simulink model "ur5_simulink_ros2_pbvs_all_methods_2023b"  (R2023b)
settings: Solver=ode4  StartTime=0.0  StopTime=inf  FixedStep=0.005  RelTol=1e-3
InitFcn:
  | l=5;
model workspace (MAT data in the model file):
  SL_ROS_VariableLengthArrays_MaxSizes : object (value not decoded)
values from neighbouring files (symbols this model uses):
  D = zeros(6,12)    [ibvs_cstate.m]
undefined symbols (not defined in the file or in its folder): data, data_SL_Info, DiscIntNeverNeededParam
libraries: simulink x9, ros2lib x8, slpidlib x6, robotmaniplib x3, mpclib x3, robotcorelib x1
(part 2 of 2)

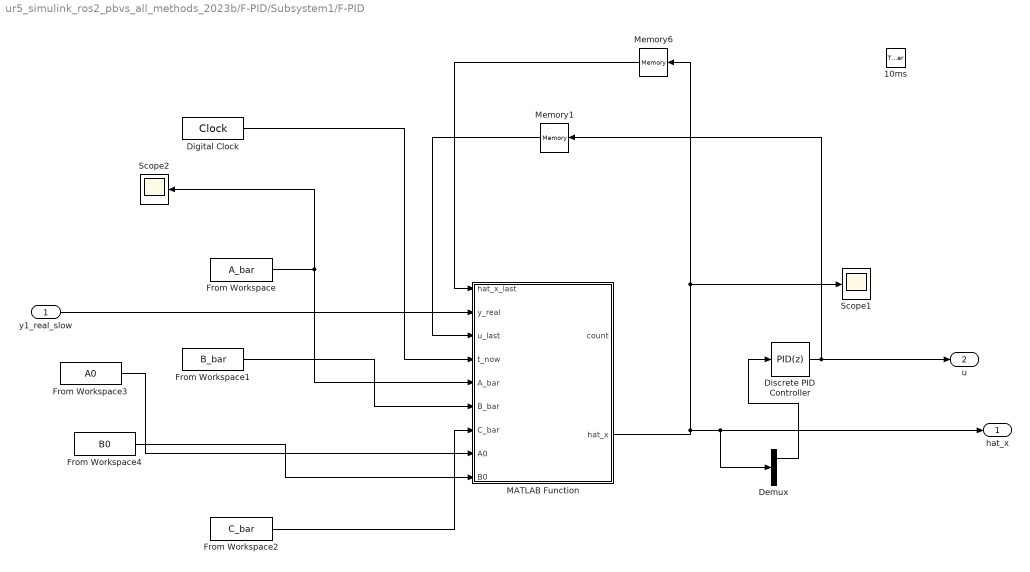
== system ur5_simulink_ros2_pbvs_all_methods_2023b/F-PID/Subsystem1/F-PID ==
  y1_real_slow : Inport
  10ms : TriggerPort  VariantControl=(inherit)  InitialTriggerSignalState=zero  PortDimensions=1
  Demux : Demux  Outputs=2
  Digital Clock : DigitalClock  SampleTime=-1
  Discrete PID Controller : slpidlib/PID Controller  Controller=PID  Form=Parallel  TimeDomain=Discrete-time  UseExternalTs=off  SampleTime=-1  IntegratorMethod=Forward Euler  FilterMethod=Forward Euler  ControllerParametersSource=internal  P=4.7  I=5  UseKiTs=off  D=0  N=100  UseFilter=on  TunerSelectOption=Transfer Function Based (PID Tuner App)  InitialConditionSource=internal  InitialConditionForIntegrator=0  InitialConditionForFilter=0  DifferentiatorICPrevScaledInput=0  ExternalReset=none  TrackingMode=off  Kt=1  LimitOutput=off  SatLimitsSource=internal  UpperSaturationLimit=inf  LowerSaturationLimit=-inf  LinearizeAsGain=off  AntiWindupMode=none  Kb=1  LimitIntegrator=off  UpperIntegratorSaturationLimit=inf  LowerIntegratorSaturationLimit=-inf  POutMin=[]  POutMax=[]  IOutMin=[]  IOutMax=[]  DOutMin=[]  DOutMax=[]  NOutMin=[]  NOutMax=[]  SumOutMin=[]  SumOutMax=[]  SaturationOutMin=[]  SaturationOutMax=[]  PParamMin=[]  PParamMax=[]  IParamMin=[]  IParamMax=[]  DParamMin=[]  DParamMax=[]  NParamMin=[]  NParamMax=[]  KbParamMin=[]  KbParamMax=[]  KtParamMin=[]  KtParamMax=[]  KbOutMin=[]  KbOutMax=[]  KtOutMin=[]  KtOutMax=[]  IntegratorOutMin=[]  IntegratorOutMax=[]  FilterOutMin=[]  FilterOutMax=[]  SumI1OutMin=[]  SumI1OutMax=[]  SumI2OutMin=[]  SumI2OutMax=[]  SumI3OutMin=[]  SumI3OutMax=[]  SumI4OutMin=[]  SumI4OutMax=[]  SumDOutMin=[]  SumDOutMax=[]  DifferentiatorOutMin=[]  DifferentiatorOutMax=[]  FilterDiffOutCoefMin=[]  FilterDiffOutCoefMax=[]  ReciprocalOutMin=[]  ReciprocalOutMax=[]  SumDenOutMin=[]  SumDenOutMax=[]  SumNumOutMin=[]  SumNumOutMax=[]  DivideOutMin=[]  DivideOutMax=[]  UdiffTsProdOutMin=[]  UdiffTsProdOutMax=[]  NTsProdOutMin=[]  NTsProdOutMax=[]  UintegralTsProdOutMin=[]  UintegralTsProdOutMax=[]  UngainTsProdOutMin=[]  UngainTsProdOutMax=[]  ClampingZeroOutDataTypeStr=Inherit: Inherit via back propagation  ClampingZeroOutMin=[]  ClampingZeroOutMax=[]  FilterDenConstantOutDataTypeStr=Inherit: Inherit via back propagation  FilterDenConstantOutMin=[]  FilterDenConstantOutMax=[]  PCopyOutDataTypeStr=Inherit: Inherit via back propagation  PCopyOutMin=[]  PCopyOutMax=[]  NCopyOutDataTypeStr=Inherit: Inherit via back propagation  NCopyOutMin=[]  NCopyOutMax=[]  IntegratorContinuousStateAttributes=''  IntegratorStateMustResolveToSignalObject=off  IntegratorRTWStateStorageClass=Auto  FilterContinuousStateAttributes=''  FilterStateMustResolveToSignalObject=off  FilterRTWStateStorageClass=Auto  ParallelPVariant=InternalParameters  IdealPVariant=Disabled  IVariant=InternalParameters  DVariant=InternalParameters  IntegratorVariant=Discrete  SatVariant=Disabled  AWVariant=Passthrough  PCopyVariant=Disabled  TRVariant=Disabled  FdbkBlocksVariant=Forward  IdealPFdbkVariant=Disabled  SatFdbkVariant=Disabled  DerivativeFilterVariant=ForwardEulerFilter  NVariant=InternalParameters  NCopyVariant=Disabled  FilterICVariant=InternalICsFilter  IntegratorICVariant=InternalICs  ExternalResetVariant=Disabled  TRSumVariant=Passthrough  SumFdbkVariant=Disabled  SumVariant=Sum_PID  TsampFilterVariant=InternalTs  TsampNgainVariant=Passthrough  TsampIntegralVariant=Disabled_SignalSpec  ExternalSaturationOutDataTypeStr=Inherit: Same as second input
      settings: LibrarySourceBlock=simulink/Discrete/Discrete PID Controller
  From Workspace : FromWorkspace  VariableName=A_bar  OutDataTypeStr=double  SampleTime=-1  OutputAfterFinalValue=Holding final value
  From Workspace1 : FromWorkspace  VariableName=B_bar  OutDataTypeStr=double  SampleTime=-1  OutputAfterFinalValue=Holding final value
  From Workspace2 : FromWorkspace  VariableName=C_bar  OutDataTypeStr=double  SampleTime=-1  OutputAfterFinalValue=Holding final value
  From Workspace3 : FromWorkspace  VariableName=A0  OutDataTypeStr=double  SampleTime=-1  OutputAfterFinalValue=Holding final value
  From Workspace4 : FromWorkspace  VariableName=B0  OutDataTypeStr=double  SampleTime=-1  OutputAfterFinalValue=Holding final value
  MATLAB Function : MATLAB Function  TreatAsAtomicUnit=on
  Memory1 : Memory  InheritSampleTime=on
  Memory6 : Memory  InheritSampleTime=on
  Scope1 : Scope
  Scope2 : Scope
  hat_x : Outport
  u : Outport  Port=2
  wires:
  From Workspace2/1 -> MATLAB Function/7(C_bar)
  From Workspace1/1 -> MATLAB Function/6(B_bar)
  Digital Clock/1 -> MATLAB Function/4(t_now)
  From Workspace/1 -> Scope2/1, MATLAB Function/5(A_bar)
  MATLAB Function/2(hat_x) -> Memory6/1, Scope1/1, Demux/1, hat_x/1
  y1_real_slow/1 -> MATLAB Function/2(y_real)
  From Workspace3/1 -> MATLAB Function/8(A0)
  From Workspace4/1 -> MATLAB Function/9(B0)
  Memory6/1 -> MATLAB Function/1(hat_x_last)
  Discrete PID Controller/1 -> Memory1/1, u/1
  Demux/1 -> Discrete PID Controller/1
  Memory1/1 -> MATLAB Function/3(u_last)

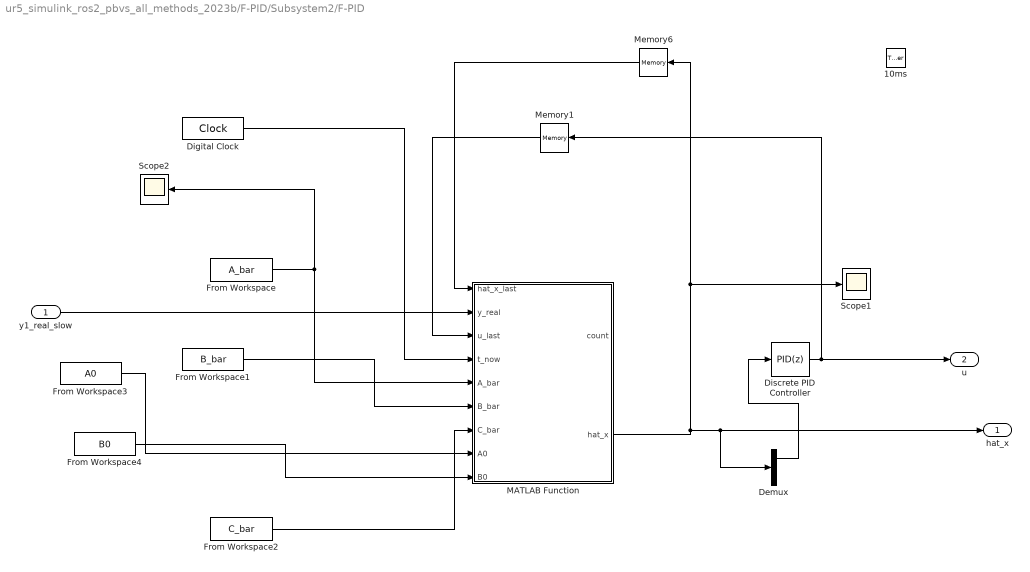
== system ur5_simulink_ros2_pbvs_all_methods_2023b/F-PID/Subsystem2/F-PID ==
  y1_real_slow : Inport
  10ms : TriggerPort  VariantControl=(inherit)  InitialTriggerSignalState=zero  PortDimensions=1
  Demux : Demux  Outputs=2
  Digital Clock : DigitalClock  SampleTime=-1
  Discrete PID Controller : slpidlib/PID Controller  Controller=PID  Form=Parallel  TimeDomain=Discrete-time  UseExternalTs=off  SampleTime=-1  IntegratorMethod=Forward Euler  FilterMethod=Forward Euler  ControllerParametersSource=internal  P=4.7  I=5  UseKiTs=off  D=0  N=100  UseFilter=on  TunerSelectOption=Transfer Function Based (PID Tuner App)  InitialConditionSource=internal  InitialConditionForIntegrator=0  InitialConditionForFilter=0  DifferentiatorICPrevScaledInput=0  ExternalReset=none  TrackingMode=off  Kt=1  LimitOutput=off  SatLimitsSource=internal  UpperSaturationLimit=inf  LowerSaturationLimit=-inf  LinearizeAsGain=off  AntiWindupMode=none  Kb=1  LimitIntegrator=off  UpperIntegratorSaturationLimit=inf  LowerIntegratorSaturationLimit=-inf  POutMin=[]  POutMax=[]  IOutMin=[]  IOutMax=[]  DOutMin=[]  DOutMax=[]  NOutMin=[]  NOutMax=[]  SumOutMin=[]  SumOutMax=[]  SaturationOutMin=[]  SaturationOutMax=[]  PParamMin=[]  PParamMax=[]  IParamMin=[]  IParamMax=[]  DParamMin=[]  DParamMax=[]  NParamMin=[]  NParamMax=[]  KbParamMin=[]  KbParamMax=[]  KtParamMin=[]  KtParamMax=[]  KbOutMin=[]  KbOutMax=[]  KtOutMin=[]  KtOutMax=[]  IntegratorOutMin=[]  IntegratorOutMax=[]  FilterOutMin=[]  FilterOutMax=[]  SumI1OutMin=[]  SumI1OutMax=[]  SumI2OutMin=[]  SumI2OutMax=[]  SumI3OutMin=[]  SumI3OutMax=[]  SumI4OutMin=[]  SumI4OutMax=[]  SumDOutMin=[]  SumDOutMax=[]  DifferentiatorOutMin=[]  DifferentiatorOutMax=[]  FilterDiffOutCoefMin=[]  FilterDiffOutCoefMax=[]  ReciprocalOutMin=[]  ReciprocalOutMax=[]  SumDenOutMin=[]  SumDenOutMax=[]  SumNumOutMin=[]  SumNumOutMax=[]  DivideOutMin=[]  DivideOutMax=[]  UdiffTsProdOutMin=[]  UdiffTsProdOutMax=[]  NTsProdOutMin=[]  NTsProdOutMax=[]  UintegralTsProdOutMin=[]  UintegralTsProdOutMax=[]  UngainTsProdOutMin=[]  UngainTsProdOutMax=[]  ClampingZeroOutDataTypeStr=Inherit: Inherit via back propagation  ClampingZeroOutMin=[]  ClampingZeroOutMax=[]  FilterDenConstantOutDataTypeStr=Inherit: Inherit via back propagation  FilterDenConstantOutMin=[]  FilterDenConstantOutMax=[]  PCopyOutDataTypeStr=Inherit: Inherit via back propagation  PCopyOutMin=[]  PCopyOutMax=[]  NCopyOutDataTypeStr=Inherit: Inherit via back propagation  NCopyOutMin=[]  NCopyOutMax=[]  IntegratorContinuousStateAttributes=''  IntegratorStateMustResolveToSignalObject=off  IntegratorRTWStateStorageClass=Auto  FilterContinuousStateAttributes=''  FilterStateMustResolveToSignalObject=off  FilterRTWStateStorageClass=Auto  ParallelPVariant=InternalParameters  IdealPVariant=Disabled  IVariant=InternalParameters  DVariant=InternalParameters  IntegratorVariant=Discrete  SatVariant=Disabled  AWVariant=Passthrough  PCopyVariant=Disabled  TRVariant=Disabled  FdbkBlocksVariant=Forward  IdealPFdbkVariant=Disabled  SatFdbkVariant=Disabled  DerivativeFilterVariant=ForwardEulerFilter  NVariant=InternalParameters  NCopyVariant=Disabled  FilterICVariant=InternalICsFilter  IntegratorICVariant=InternalICs  ExternalResetVariant=Disabled  TRSumVariant=Passthrough  SumFdbkVariant=Disabled  SumVariant=Sum_PID  TsampFilterVariant=InternalTs  TsampNgainVariant=Passthrough  TsampIntegralVariant=Disabled_SignalSpec  ExternalSaturationOutDataTypeStr=Inherit: Same as second input
      settings: LibrarySourceBlock=simulink/Discrete/Discrete PID Controller
  From Workspace : FromWorkspace  VariableName=A_bar  OutDataTypeStr=double  SampleTime=-1  OutputAfterFinalValue=Holding final value
  From Workspace1 : FromWorkspace  VariableName=B_bar  OutDataTypeStr=double  SampleTime=-1  OutputAfterFinalValue=Holding final value
  From Workspace2 : FromWorkspace  VariableName=C_bar  OutDataTypeStr=double  SampleTime=-1  OutputAfterFinalValue=Holding final value
  From Workspace3 : FromWorkspace  VariableName=A0  OutDataTypeStr=double  SampleTime=-1  OutputAfterFinalValue=Holding final value
  From Workspace4 : FromWorkspace  VariableName=B0  OutDataTypeStr=double  SampleTime=-1  OutputAfterFinalValue=Holding final value
  MATLAB Function : MATLAB Function  TreatAsAtomicUnit=on
  Memory1 : Memory  InheritSampleTime=on
  Memory6 : Memory  InheritSampleTime=on
  Scope1 : Scope
  Scope2 : Scope
  hat_x : Outport
  u : Outport  Port=2
  wires:
  From Workspace2/1 -> MATLAB Function/7(C_bar)
  From Workspace1/1 -> MATLAB Function/6(B_bar)
  Digital Clock/1 -> MATLAB Function/4(t_now)
  From Workspace/1 -> Scope2/1, MATLAB Function/5(A_bar)
  MATLAB Function/2(hat_x) -> Memory6/1, Scope1/1, Demux/1, hat_x/1
  y1_real_slow/1 -> MATLAB Function/2(y_real)
  From Workspace3/1 -> MATLAB Function/8(A0)
  From Workspace4/1 -> MATLAB Function/9(B0)
  Memory6/1 -> MATLAB Function/1(hat_x_last)
  Discrete PID Controller/1 -> Memory1/1, u/1
  Demux/1 -> Discrete PID Controller/1
  Memory1/1 -> MATLAB Function/3(u_last)

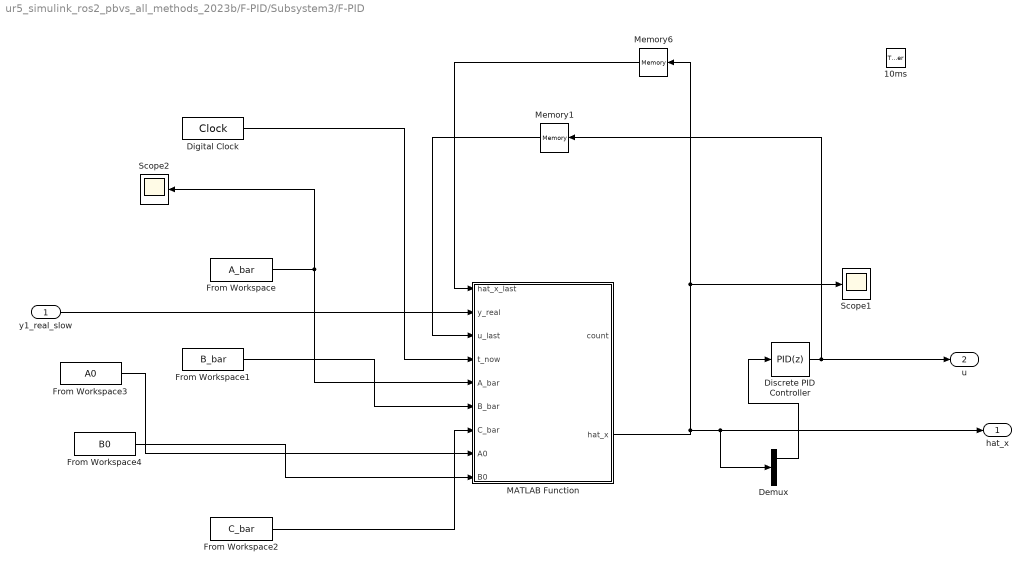
== system ur5_simulink_ros2_pbvs_all_methods_2023b/F-PID/Subsystem3/F-PID ==
  y1_real_slow : Inport
  10ms : TriggerPort  VariantControl=(inherit)  InitialTriggerSignalState=zero  PortDimensions=1
  Demux : Demux  Outputs=2
  Digital Clock : DigitalClock  SampleTime=-1
  Discrete PID Controller : slpidlib/PID Controller  Controller=PID  Form=Parallel  TimeDomain=Discrete-time  UseExternalTs=off  SampleTime=-1  IntegratorMethod=Forward Euler  FilterMethod=Forward Euler  ControllerParametersSource=internal  P=4.7  I=5  UseKiTs=off  D=0  N=100  UseFilter=on  TunerSelectOption=Transfer Function Based (PID Tuner App)  InitialConditionSource=internal  InitialConditionForIntegrator=0  InitialConditionForFilter=0  DifferentiatorICPrevScaledInput=0  ExternalReset=none  TrackingMode=off  Kt=1  LimitOutput=off  SatLimitsSource=internal  UpperSaturationLimit=inf  LowerSaturationLimit=-inf  LinearizeAsGain=off  AntiWindupMode=none  Kb=1  LimitIntegrator=off  UpperIntegratorSaturationLimit=inf  LowerIntegratorSaturationLimit=-inf  POutMin=[]  POutMax=[]  IOutMin=[]  IOutMax=[]  DOutMin=[]  DOutMax=[]  NOutMin=[]  NOutMax=[]  SumOutMin=[]  SumOutMax=[]  SaturationOutMin=[]  SaturationOutMax=[]  PParamMin=[]  PParamMax=[]  IParamMin=[]  IParamMax=[]  DParamMin=[]  DParamMax=[]  NParamMin=[]  NParamMax=[]  KbParamMin=[]  KbParamMax=[]  KtParamMin=[]  KtParamMax=[]  KbOutMin=[]  KbOutMax=[]  KtOutMin=[]  KtOutMax=[]  IntegratorOutMin=[]  IntegratorOutMax=[]  FilterOutMin=[]  FilterOutMax=[]  SumI1OutMin=[]  SumI1OutMax=[]  SumI2OutMin=[]  SumI2OutMax=[]  SumI3OutMin=[]  SumI3OutMax=[]  SumI4OutMin=[]  SumI4OutMax=[]  SumDOutMin=[]  SumDOutMax=[]  DifferentiatorOutMin=[]  DifferentiatorOutMax=[]  FilterDiffOutCoefMin=[]  FilterDiffOutCoefMax=[]  ReciprocalOutMin=[]  ReciprocalOutMax=[]  SumDenOutMin=[]  SumDenOutMax=[]  SumNumOutMin=[]  SumNumOutMax=[]  DivideOutMin=[]  DivideOutMax=[]  UdiffTsProdOutMin=[]  UdiffTsProdOutMax=[]  NTsProdOutMin=[]  NTsProdOutMax=[]  UintegralTsProdOutMin=[]  UintegralTsProdOutMax=[]  UngainTsProdOutMin=[]  UngainTsProdOutMax=[]  ClampingZeroOutDataTypeStr=Inherit: Inherit via back propagation  ClampingZeroOutMin=[]  ClampingZeroOutMax=[]  FilterDenConstantOutDataTypeStr=Inherit: Inherit via back propagation  FilterDenConstantOutMin=[]  FilterDenConstantOutMax=[]  PCopyOutDataTypeStr=Inherit: Inherit via back propagation  PCopyOutMin=[]  PCopyOutMax=[]  NCopyOutDataTypeStr=Inherit: Inherit via back propagation  NCopyOutMin=[]  NCopyOutMax=[]  IntegratorContinuousStateAttributes=''  IntegratorStateMustResolveToSignalObject=off  IntegratorRTWStateStorageClass=Auto  FilterContinuousStateAttributes=''  FilterStateMustResolveToSignalObject=off  FilterRTWStateStorageClass=Auto  ParallelPVariant=InternalParameters  IdealPVariant=Disabled  IVariant=InternalParameters  DVariant=InternalParameters  IntegratorVariant=Discrete  SatVariant=Disabled  AWVariant=Passthrough  PCopyVariant=Disabled  TRVariant=Disabled  FdbkBlocksVariant=Forward  IdealPFdbkVariant=Disabled  SatFdbkVariant=Disabled  DerivativeFilterVariant=ForwardEulerFilter  NVariant=InternalParameters  NCopyVariant=Disabled  FilterICVariant=InternalICsFilter  IntegratorICVariant=InternalICs  ExternalResetVariant=Disabled  TRSumVariant=Passthrough  SumFdbkVariant=Disabled  SumVariant=Sum_PID  TsampFilterVariant=InternalTs  TsampNgainVariant=Passthrough  TsampIntegralVariant=Disabled_SignalSpec  ExternalSaturationOutDataTypeStr=Inherit: Same as second input
      settings: LibrarySourceBlock=simulink/Discrete/Discrete PID Controller
  From Workspace : FromWorkspace  VariableName=A_bar  OutDataTypeStr=double  SampleTime=-1  OutputAfterFinalValue=Holding final value
  From Workspace1 : FromWorkspace  VariableName=B_bar  OutDataTypeStr=double  SampleTime=-1  OutputAfterFinalValue=Holding final value
  From Workspace2 : FromWorkspace  VariableName=C_bar  OutDataTypeStr=double  SampleTime=-1  OutputAfterFinalValue=Holding final value
  From Workspace3 : FromWorkspace  VariableName=A0  OutDataTypeStr=double  SampleTime=-1  OutputAfterFinalValue=Holding final value
  From Workspace4 : FromWorkspace  VariableName=B0  OutDataTypeStr=double  SampleTime=-1  OutputAfterFinalValue=Holding final value
  MATLAB Function : MATLAB Function  TreatAsAtomicUnit=on
  Memory1 : Memory  InheritSampleTime=on
  Memory6 : Memory  InheritSampleTime=on
  Scope1 : Scope
  Scope2 : Scope
  hat_x : Outport
  u : Outport  Port=2
  wires:
  From Workspace2/1 -> MATLAB Function/7(C_bar)
  From Workspace1/1 -> MATLAB Function/6(B_bar)
  Digital Clock/1 -> MATLAB Function/4(t_now)
  From Workspace/1 -> Scope2/1, MATLAB Function/5(A_bar)
  MATLAB Function/2(hat_x) -> Memory6/1, Scope1/1, Demux/1, hat_x/1
  y1_real_slow/1 -> MATLAB Function/2(y_real)
  From Workspace3/1 -> MATLAB Function/8(A0)
  From Workspace4/1 -> MATLAB Function/9(B0)
  Memory6/1 -> MATLAB Function/1(hat_x_last)
  Discrete PID Controller/1 -> Memory1/1, u/1
  Demux/1 -> Discrete PID Controller/1
  Memory1/1 -> MATLAB Function/3(u_last)

== system ur5_simulink_ros2_pbvs_all_methods_2023b/MPC-DOB/mpc/Subsystem ==
  ex : Inport
  u : Inport  Port=2
  Trigger : TriggerPort  VariantControl=(inherit)  PortDimensions=1
  Scope : Scope
  Scope5 : Scope
  dob : Subsystem
  dhat : Outport
  wires:
  ex/1 -> Scope/1, dob/1(ex)
  dob/1(dhat) -> dhat/1, Scope5/1
  u/1 -> dob/2(u)

== system ur5_simulink_ros2_pbvs_all_methods_2023b/MPC-DOB/mpc1/Subsystem ==
  ex : Inport
  u : Inport  Port=2
  Trigger : TriggerPort  VariantControl=(inherit)  PortDimensions=1
  Scope : Scope
  Scope5 : Scope
  dob : Subsystem
  dhat : Outport
  wires:
  ex/1 -> Scope/1, dob/1(ex)
  dob/1(dhat) -> dhat/1, Scope5/1
  u/1 -> dob/2(u)

== system ur5_simulink_ros2_pbvs_all_methods_2023b/MPC-DOB/mpc2/Subsystem ==
  ex : Inport
  u : Inport  Port=2
  Trigger : TriggerPort  VariantControl=(inherit)  PortDimensions=1
  Scope : Scope
  Scope5 : Scope
  dob : Subsystem
  dhat : Outport
  wires:
  ex/1 -> Scope/1, dob/1(ex)
  dob/1(dhat) -> dhat/1, Scope5/1
  u/1 -> dob/2(u)

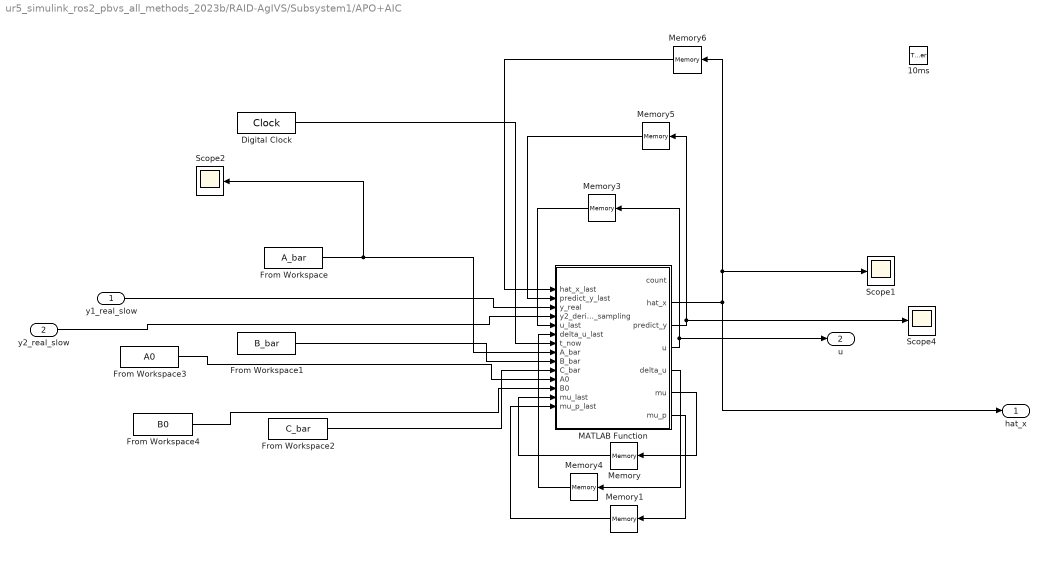
== system ur5_simulink_ros2_pbvs_all_methods_2023b/RAID-AgIVS/Subsystem1/APO+AIC ==
  y1_real_slow : Inport
  y2_real_slow : Inport  Port=2
  10ms : TriggerPort  VariantControl=(inherit)  InitialTriggerSignalState=zero  PortDimensions=1
  Digital Clock : DigitalClock  SampleTime=-1
  From Workspace : FromWorkspace  VariableName=A_bar  OutDataTypeStr=double  SampleTime=-1  OutputAfterFinalValue=Holding final value
  From Workspace1 : FromWorkspace  VariableName=B_bar  OutDataTypeStr=double  SampleTime=-1  OutputAfterFinalValue=Holding final value
  From Workspace2 : FromWorkspace  VariableName=C_bar  OutDataTypeStr=double  SampleTime=-1  OutputAfterFinalValue=Holding final value
  From Workspace3 : FromWorkspace  VariableName=A0  OutDataTypeStr=double  SampleTime=-1  OutputAfterFinalValue=Holding final value
  From Workspace4 : FromWorkspace  VariableName=B0  OutDataTypeStr=double  SampleTime=-1  OutputAfterFinalValue=Holding final value
  MATLAB Function : MATLAB Function  TreatAsAtomicUnit=on
  Memory{,1,3..6} (6 alike) : Memory  InheritSampleTime=on
  Scope1 : Scope
  Scope2 : Scope
  Scope4 : Scope
  hat_x : Outport
  u : Outport  Port=2
  wires:
  From Workspace2/1 -> MATLAB Function/10(C_bar)
  From Workspace1/1 -> MATLAB Function/9(B_bar)
  Digital Clock/1 -> MATLAB Function/7(t_now)
  Memory5/1 -> MATLAB Function/2(predict_y_last)
  MATLAB Function/3(predict_y) -> Memory5/1, Scope4/1
  From Workspace/1 -> Scope2/1, MATLAB Function/8(A_bar)
  MATLAB Function/2(hat_x) -> Memory6/1, Scope1/1, hat_x/1
  y1_real_slow/1 -> MATLAB Function/3(y_real)
  From Workspace3/1 -> MATLAB Function/11(A0)
  From Workspace4/1 -> MATLAB Function/12(B0)
  MATLAB Function/6(mu) -> Memory/1
  Memory/1 -> MATLAB Function/13(mu_last)
  MATLAB Function/7(mu_p) -> Memory1/1
  Memory1/1 -> MATLAB Function/14(mu_p_last)
  y2_real_slow/1 -> MATLAB Function/4(y2_derivative_sampling)
  MATLAB Function/4(u) -> Memory3/1, u/1
  Memory3/1 -> MATLAB Function/5(u_last)
  MATLAB Function/5(delta_u) -> Memory4/1
  Memory6/1 -> MATLAB Function/1(hat_x_last)
  Memory4/1 -> MATLAB Function/6(delta_u_last)

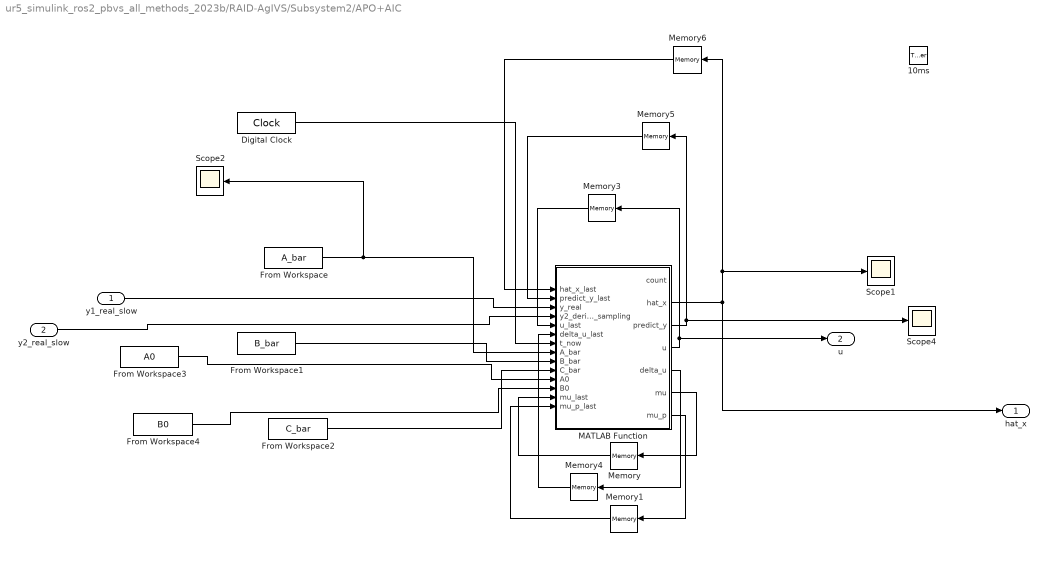
== system ur5_simulink_ros2_pbvs_all_methods_2023b/RAID-AgIVS/Subsystem2/APO+AIC ==
  y1_real_slow : Inport
  y2_real_slow : Inport  Port=2
  10ms : TriggerPort  VariantControl=(inherit)  InitialTriggerSignalState=zero  PortDimensions=1
  Digital Clock : DigitalClock  SampleTime=-1
  From Workspace : FromWorkspace  VariableName=A_bar  OutDataTypeStr=double  SampleTime=-1  OutputAfterFinalValue=Holding final value
  From Workspace1 : FromWorkspace  VariableName=B_bar  OutDataTypeStr=double  SampleTime=-1  OutputAfterFinalValue=Holding final value
  From Workspace2 : FromWorkspace  VariableName=C_bar  OutDataTypeStr=double  SampleTime=-1  OutputAfterFinalValue=Holding final value
  From Workspace3 : FromWorkspace  VariableName=A0  OutDataTypeStr=double  SampleTime=-1  OutputAfterFinalValue=Holding final value
  From Workspace4 : FromWorkspace  VariableName=B0  OutDataTypeStr=double  SampleTime=-1  OutputAfterFinalValue=Holding final value
  MATLAB Function : MATLAB Function  TreatAsAtomicUnit=on
  Memory{,1,3..6} (6 alike) : Memory  InheritSampleTime=on
  Scope1 : Scope
  Scope2 : Scope
  Scope4 : Scope
  hat_x : Outport
  u : Outport  Port=2
  wires:
  From Workspace2/1 -> MATLAB Function/10(C_bar)
  From Workspace1/1 -> MATLAB Function/9(B_bar)
  Digital Clock/1 -> MATLAB Function/7(t_now)
  Memory5/1 -> MATLAB Function/2(predict_y_last)
  MATLAB Function/3(predict_y) -> Memory5/1, Scope4/1
  From Workspace/1 -> Scope2/1, MATLAB Function/8(A_bar)
  MATLAB Function/2(hat_x) -> Memory6/1, Scope1/1, hat_x/1
  y1_real_slow/1 -> MATLAB Function/3(y_real)
  From Workspace3/1 -> MATLAB Function/11(A0)
  From Workspace4/1 -> MATLAB Function/12(B0)
  MATLAB Function/6(mu) -> Memory/1
  Memory/1 -> MATLAB Function/13(mu_last)
  MATLAB Function/7(mu_p) -> Memory1/1
  Memory1/1 -> MATLAB Function/14(mu_p_last)
  y2_real_slow/1 -> MATLAB Function/4(y2_derivative_sampling)
  MATLAB Function/4(u) -> Memory3/1, u/1
  Memory3/1 -> MATLAB Function/5(u_last)
  MATLAB Function/5(delta_u) -> Memory4/1
  Memory6/1 -> MATLAB Function/1(hat_x_last)
  Memory4/1 -> MATLAB Function/6(delta_u_last)

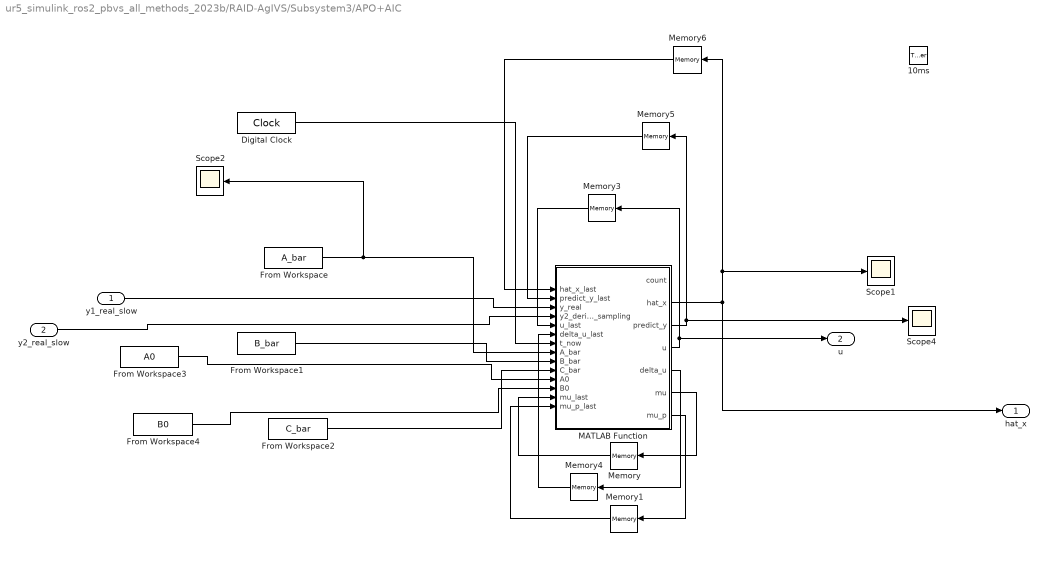
== system ur5_simulink_ros2_pbvs_all_methods_2023b/RAID-AgIVS/Subsystem3/APO+AIC ==
  y1_real_slow : Inport
  y2_real_slow : Inport  Port=2
  10ms : TriggerPort  VariantControl=(inherit)  InitialTriggerSignalState=zero  PortDimensions=1
  Digital Clock : DigitalClock  SampleTime=-1
  From Workspace : FromWorkspace  VariableName=A_bar  OutDataTypeStr=double  SampleTime=-1  OutputAfterFinalValue=Holding final value
  From Workspace1 : FromWorkspace  VariableName=B_bar  OutDataTypeStr=double  SampleTime=-1  OutputAfterFinalValue=Holding final value
  From Workspace2 : FromWorkspace  VariableName=C_bar  OutDataTypeStr=double  SampleTime=-1  OutputAfterFinalValue=Holding final value
  From Workspace3 : FromWorkspace  VariableName=A0  OutDataTypeStr=double  SampleTime=-1  OutputAfterFinalValue=Holding final value
  From Workspace4 : FromWorkspace  VariableName=B0  OutDataTypeStr=double  SampleTime=-1  OutputAfterFinalValue=Holding final value
  MATLAB Function : MATLAB Function  TreatAsAtomicUnit=on
  Memory{,1,3..6} (6 alike) : Memory  InheritSampleTime=on
  Scope1 : Scope
  Scope2 : Scope
  Scope4 : Scope
  hat_x : Outport
  u : Outport  Port=2
  wires:
  From Workspace2/1 -> MATLAB Function/10(C_bar)
  From Workspace1/1 -> MATLAB Function/9(B_bar)
  Digital Clock/1 -> MATLAB Function/7(t_now)
  Memory5/1 -> MATLAB Function/2(predict_y_last)
  MATLAB Function/3(predict_y) -> Memory5/1, Scope4/1
  From Workspace/1 -> Scope2/1, MATLAB Function/8(A_bar)
  MATLAB Function/2(hat_x) -> Memory6/1, Scope1/1, hat_x/1
  y1_real_slow/1 -> MATLAB Function/3(y_real)
  From Workspace3/1 -> MATLAB Function/11(A0)
  From Workspace4/1 -> MATLAB Function/12(B0)
  MATLAB Function/6(mu) -> Memory/1
  Memory/1 -> MATLAB Function/13(mu_last)
  MATLAB Function/7(mu_p) -> Memory1/1
  Memory1/1 -> MATLAB Function/14(mu_p_last)
  y2_real_slow/1 -> MATLAB Function/4(y2_derivative_sampling)
  MATLAB Function/4(u) -> Memory3/1, u/1
  Memory3/1 -> MATLAB Function/5(u_last)
  MATLAB Function/5(delta_u) -> Memory4/1
  Memory6/1 -> MATLAB Function/1(hat_x_last)
  Memory4/1 -> MATLAB Function/6(delta_u_last)

== system ur5_simulink_ros2_pbvs_all_methods_2023b/MPC-DOB/mpc/Subsystem/dob ==
  ex : Inport
  u : Inport  Port=2
  Add3 : Sum
  Add4 : Sum  Inputs=+-
  Discrete-Time Integrator : DiscreteIntegrator  SampleTime=-1  LimitOutput=on  UpperSaturationLimit=5  LowerSaturationLimit=-5  ICPrevOutput=DiscIntNeverNeededParam  ICPrevScaledInput=DiscIntNeverNeededParam
  Gain1 : Gain  Gain=-l
  Gain2 : Gain  Gain=l
  dhat : Outport
  wires:
  Gain1/1 -> Discrete-Time Integrator/1
  Add4/1 -> Gain1/1
  Add3/1 -> dhat/1, Add4/1
  Gain2/1 -> Add3/1
  Discrete-Time Integrator/1 -> Add3/2
  ex/1 -> Gain2/1
  u/1 -> Add4/2

== system ur5_simulink_ros2_pbvs_all_methods_2023b/MPC-DOB/mpc1/Subsystem/dob ==
  ex : Inport
  u : Inport  Port=2
  Add3 : Sum
  Add4 : Sum  Inputs=+-
  Discrete-Time Integrator : DiscreteIntegrator  SampleTime=-1  LimitOutput=on  UpperSaturationLimit=5  LowerSaturationLimit=-5  ICPrevOutput=DiscIntNeverNeededParam  ICPrevScaledInput=DiscIntNeverNeededParam
  Gain1 : Gain  Gain=-l
  Gain2 : Gain  Gain=l
  dhat : Outport
  wires:
  Gain1/1 -> Discrete-Time Integrator/1
  Add4/1 -> Gain1/1
  Add3/1 -> dhat/1, Add4/1
  Gain2/1 -> Add3/1
  Discrete-Time Integrator/1 -> Add3/2
  ex/1 -> Gain2/1
  u/1 -> Add4/2

== system ur5_simulink_ros2_pbvs_all_methods_2023b/MPC-DOB/mpc2/Subsystem/dob ==
  ex : Inport
  u : Inport  Port=2
  Add3 : Sum
  Add4 : Sum  Inputs=+-
  Discrete-Time Integrator : DiscreteIntegrator  SampleTime=-1  LimitOutput=on  UpperSaturationLimit=5  LowerSaturationLimit=-5  ICPrevOutput=DiscIntNeverNeededParam  ICPrevScaledInput=DiscIntNeverNeededParam
  Gain1 : Gain  Gain=-l
  Gain2 : Gain  Gain=l
  dhat : Outport
  wires:
  Gain1/1 -> Discrete-Time Integrator/1
  Add4/1 -> Gain1/1
  Add3/1 -> dhat/1, Add4/1
  Gain2/1 -> Add3/1
  Discrete-Time Integrator/1 -> Add3/2
  ex/1 -> Gain2/1
  u/1 -> Add4/2

== matlab function ur5_simulink_ros2_pbvs_all_methods_2023b/F-PID/Subsystem1/F-PID/MATLAB Function ==
  data: count output; hat_x_last input; y_real input; u_last input; hat_x output; t_now input; A_bar input; B_bar input; C_bar input; A0 input; B0 input
function [count, hat_x] = fcn(hat_x_last, y_real, u_last, t_now,A_bar,B_bar,C_bar,A0,B0)
if(t_now==0)
    count=0;
    hat_x = zeros(2,1);
    hat_x(1,1)=y_real;
else
    count=mod(t_now,0.05);
    if(count==0)%在采样的时刻
        hat_x=A_bar*hat_x_last +B_bar*u_last+ C_bar*y_real;
    else%在两个采样时刻之间
        hat_x = A0*hat_x_last+B0*u_last;
    end
end
end

% function [count,hat_x,predict_y, u, delta_u, mu, mu_p, mu_pp] = fcn(hat_x_last, predict_y_last, y_real,y2_derivative_sampling,y3_real_slow, u_last,delta_u_last,t_now,A_bar,B_bar,C_bar,A0,B0,mu_last, mu_p_last, mu_pp_last)
% if(t_now==0)
%     count=0;
%     hat_x = zeros(3,1);
%     predict_y = y_real;
%     hat_x(1,1)=y_real;
%     u_now=0;
%     hat_x = A_bar*hat_x + B_bar*u_now+ C_bar*predict_y;
%     [u, delta_u, mu, mu_p, mu_pp]  = AIC3(t_now, 1, y_real,hat_x(1,1),y2_derivative_sampling,hat_x(2,1), y3_real_slow, hat_x(3,1), mu_last, mu_p_last, mu_pp_last, u_last);
%     %predict_y=[1 0 0]*(A0*hat_x+B0*delta_u); 
%     
% else
%     count=mod(t_now,0.05);
%     if(count==0)%在采样的时刻
%         predict_y=y_real;
%         hat_x=A_bar*hat_x_last +B_bar*delta_u_last+ C_bar*predict_y;
%         %hat_x(1,1)=y_real;
%         [u, delta_u, mu, mu_p, mu_pp]  = AIC3(t_now, 1, y_real,hat_x(1,1),y2_derivative_sampling,hat_x(2,1), y3_real_slow, hat_x(3,1), mu_last, mu_p_last, mu_pp_last, u_last);
% 
%         %predict_y=[1 0 0]*(A0*hat_x+B0*delta_u);
%         
%     else%在两个采样时刻之间
%         predict_y=[1 0 0]*(A0*hat_x_last+B0*delta_u_last);
%         hat_x=A_bar*hat_x_last + B_bar*delta_u_last+C_bar*predict_y_last;
%         [u, delta_u, mu, mu_p, mu_pp]  = AIC3(t_now, 1, y_real,hat_x(1,1),y2_derivative_sampling,hat_x(2,1), y3_real_slow, hat_x(3,1), mu_last, mu_p_last, mu_pp_last, u_last);
%         %predict_y=[1 0 0]*(A0*hat_x+B0*delta_u);
%         
%     end
% end
% end

== matlab function ur5_simulink_ros2_pbvs_all_methods_2023b/F-PID/Subsystem2/F-PID/MATLAB Function ==
  data: count output; hat_x_last input; y_real input; u_last input; hat_x output; t_now input; A_bar input; B_bar input; C_bar input; A0 input; B0 input
function [count, hat_x] = fcn(hat_x_last, y_real, u_last, t_now,A_bar,B_bar,C_bar,A0,B0)
if(t_now==0)
    count=0;
    hat_x = zeros(2,1);
    hat_x(1,1)=y_real;
else
    count=mod(t_now,0.05);
    if(count==0)%在采样的时刻
        hat_x=A_bar*hat_x_last +B_bar*u_last+ C_bar*y_real;
    else%在两个采样时刻之间
        hat_x = A0*hat_x_last+B0*u_last;
    end
end
end

% function [count,hat_x,predict_y, u, delta_u, mu, mu_p, mu_pp] = fcn(hat_x_last, predict_y_last, y_real,y2_derivative_sampling,y3_real_slow, u_last,delta_u_last,t_now,A_bar,B_bar,C_bar,A0,B0,mu_last, mu_p_last, mu_pp_last)
% if(t_now==0)
%     count=0;
%     hat_x = zeros(3,1);
%     predict_y = y_real;
%     hat_x(1,1)=y_real;
%     u_now=0;
%     hat_x = A_bar*hat_x + B_bar*u_now+ C_bar*predict_y;
%     [u, delta_u, mu, mu_p, mu_pp]  = AIC3(t_now, 1, y_real,hat_x(1,1),y2_derivative_sampling,hat_x(2,1), y3_real_slow, hat_x(3,1), mu_last, mu_p_last, mu_pp_last, u_last);
%     %predict_y=[1 0 0]*(A0*hat_x+B0*delta_u); 
%     
% else
%     count=mod(t_now,0.05);
%     if(count==0)%在采样的时刻
%         predict_y=y_real;
%         hat_x=A_bar*hat_x_last +B_bar*delta_u_last+ C_bar*predict_y;
%         %hat_x(1,1)=y_real;
%         [u, delta_u, mu, mu_p, mu_pp]  = AIC3(t_now, 1, y_real,hat_x(1,1),y2_derivative_sampling,hat_x(2,1), y3_real_slow, hat_x(3,1), mu_last, mu_p_last, mu_pp_last, u_last);
% 
%         %predict_y=[1 0 0]*(A0*hat_x+B0*delta_u);
%         
%     else%在两个采样时刻之间
%         predict_y=[1 0 0]*(A0*hat_x_last+B0*delta_u_last);
%         hat_x=A_bar*hat_x_last + B_bar*delta_u_last+C_bar*predict_y_last;
%         [u, delta_u, mu, mu_p, mu_pp]  = AIC3(t_now, 1, y_real,hat_x(1,1),y2_derivative_sampling,hat_x(2,1), y3_real_slow, hat_x(3,1), mu_last, mu_p_last, mu_pp_last, u_last);
%         %predict_y=[1 0 0]*(A0*hat_x+B0*delta_u);
%         
%     end
% end
% end

== matlab function ur5_simulink_ros2_pbvs_all_methods_2023b/MATLAB Function3 ==
  data: camera_rot input; obj_pos input; y output
function y = fcn(camera_rot, obj_pos)
    temp_pos = [obj_pos(1);obj_pos(2);obj_pos(3);1];
    new_pos = camera_rot*temp_pos;
    y = new_pos(1:3);
end

== matlab function ur5_simulink_ros2_pbvs_all_methods_2023b/joint vel to ros3/to ros2 ==
  data: u input; flag input; y output; joint1 input; joint2 input; joint3 input; joint4 input; joint5 input; joint6 input
function y  = fcn(u,flag, joint1, joint2, joint3, joint4, joint5, joint6)
    y = zeros(128,1);
    if(flag==0)
        y(1) = u(1);
        y(2) = u(2);
        y(3) = u(3);
        y(4) = u(4);
        y(5) = u(5);
        y(6) = u(6);
    else
        y(1) = joint1;
        y(2) = joint2;
        y(3) = joint3;
        y(4) = joint4;
        y(5) = joint5;
        y(6) = joint6;
    end
end

== matlab function ur5_simulink_ros2_pbvs_all_methods_2023b/RAID-AgIVS/Subsystem1/APO+AIC/MATLAB Function ==
  data: count output; hat_x_last input; predict_y_last input; y_real input; y2_derivative_sampling input; u_last input; delta_u_last input; hat_x output; t_now input; A_bar input; B_bar input; C_bar input; predict_y output; A0 input; B0 input; mu_last input; mu_p_last input; u output; delta_u output; mu output; mu_p output
function [count,hat_x,predict_y, u, delta_u, mu, mu_p] = fcn(hat_x_last, predict_y_last, y_real,y2_derivative_sampling, u_last,delta_u_last,t_now,A_bar,B_bar,C_bar,A0,B0,mu_last, mu_p_last)
if(t_now==0)
    count=0;
    hat_x = zeros(2,1);
    predict_y = y_real;
    hat_x(1,1)=y_real;
    [u, delta_u, mu, mu_p]  = AIC2(t_now, 1, y_real,hat_x(1,1),y2_derivative_sampling,hat_x(2,1), mu_last, mu_p_last, u_last);
else
    count=mod(t_now,0.05);
    if(count==0)%在采样的时刻
        predict_y=y_real;
        hat_x=A_bar*hat_x_last +B_bar*delta_u_last/0.01+ C_bar*predict_y;
        [u, delta_u, mu, mu_p]  = AIC2(t_now, 1, y_real,hat_x(1,1),y2_derivative_sampling,hat_x(2,1), mu_last, mu_p_last, u_last);
    else%在两个采样时刻之间
        predict_y=[1 0]*(A0*hat_x_last+B0*delta_u_last);
        hat_x=A_bar*hat_x_last + B_bar*delta_u_last/0.01+C_bar*predict_y_last;
        [u, delta_u, mu, mu_p]  = AIC2(t_now, 1, y_real,hat_x(1,1),y2_derivative_sampling,hat_x(2,1), mu_last, mu_p_last, u_last);
    end
end
end








% function [count,hat_x,predict_y, u, delta_u, mu, mu_p, mu_pp] = fcn(hat_x_last, predict_y_last, y_real,y2_derivative_sampling,y3_real_slow, u_last,delta_u_last,t_now,A_bar,B_bar,C_bar,A0,B0,mu_last, mu_p_last, mu_pp_last)
% if(t_now==0)
%     count=0;
%     hat_x = zeros(3,1);
%     predict_y = y_real;
%     hat_x(1,1)=y_real;
%     u_now=0;
%     hat_x = A_bar*hat_x + B_bar*u_now+ C_bar*predict_y;
%     [u, delta_u, mu, mu_p, mu_pp]  = AIC3(t_now, 1, y_real,hat_x(1,1),y2_derivative_sampling,hat_x(2,1), y3_real_slow, hat_x(3,1), mu_last, mu_p_last, mu_pp_last, u_last);
%     %predict_y=[1 0 0]*(A0*hat_x+B0*delta_u); 
%     
% else
%     count=mod(t_now,0.05);
%     if(count==0)%在采样的时刻
%         predict_y=y_real;
%         hat_x=A_bar*hat_x_last +B_bar*delta_u_last+ C_bar*predict_y;
%         %hat_x(1,1)=y_real;
%         [u, delta_u, mu, mu_p, mu_pp]  = AIC3(t_now, 1, y_real,hat_x(1,1),y2_derivative_sampling,hat_x(2,1), y3_real_slow, hat_x(3,1), mu_last, mu_p_last, mu_pp_last, u_last);
% 
%         %predict_y=[1 0 0]*(A0*hat_x+B0*delta_u);
%         
%     else%在两个采样时刻之间
%         predict_y=[1 0 0]*(A0*hat_x_last+B0*delta_u_last);
%         hat_x=A_bar*hat_x_last + B_bar*delta_u_last+C_bar*predict_y_last;
%         [u, delta_u, mu, mu_p, mu_pp]  = AIC3(t_now, 1, y_real,hat_x(1,1),y2_derivative_sampling,hat_x(2,1), y3_real_slow, hat_x(3,1), mu_last, mu_p_last, mu_pp_last, u_last);
%         %predict_y=[1 0 0]*(A0*hat_x+B0*delta_u);
%         
%     end
% end
% end

== matlab function ur5_simulink_ros2_pbvs_all_methods_2023b/norm jacobian ==
  data: u input; y output size=[6,6]
function y = fcn(u)
firstThreeColumns =u(1:3, :);
lastThreeColumns = u(4:6, :);
y = [lastThreeColumns;firstThreeColumns];

== matlab function ur5_simulink_ros2_pbvs_all_methods_2023b/Subsystem3/MATLAB Function ==
  data: u input; joint1_pos output; joint2_pos output; joint3_pos output; joint4_pos output; joint5_pos output; joint6_pos output
function [joint1_pos,joint2_pos,joint3_pos,joint4_pos,joint5_pos,joint6_pos] = fcn(u)
joint1_pos = u(6);
joint2_pos = u(1);
joint3_pos = u(2);
joint4_pos = u(3);
joint5_pos = u(4);
joint6_pos = u(5);

== matlab function ur5_simulink_ros2_pbvs_all_methods_2023b/RAID-AgIVS/Subsystem2/APO+AIC/MATLAB Function ==
  data: count output; hat_x_last input; predict_y_last input; y_real input; y2_derivative_sampling input; u_last input; delta_u_last input; hat_x output; t_now input; A_bar input; B_bar input; C_bar input; predict_y output; A0 input; B0 input; mu_last input; mu_p_last input; u output; delta_u output; mu output; mu_p output
function [count,hat_x,predict_y, u, delta_u, mu, mu_p] = fcn(hat_x_last, predict_y_last, y_real,y2_derivative_sampling, u_last,delta_u_last,t_now,A_bar,B_bar,C_bar,A0,B0,mu_last, mu_p_last)
if(t_now==0)
    count=0;
    hat_x = zeros(2,1);
    predict_y = y_real;
    hat_x(1,1)=y_real;
    [u, delta_u, mu, mu_p]  = AIC2(t_now, 1, y_real,hat_x(1,1),y2_derivative_sampling,hat_x(2,1), mu_last, mu_p_last, u_last);
else
    count=mod(t_now,0.05);
    if(count==0)%在采样的时刻
        predict_y=y_real;
        hat_x=A_bar*hat_x_last +B_bar*delta_u_last/0.01+ C_bar*predict_y;
        [u, delta_u, mu, mu_p]  = AIC2(t_now, 1, y_real,hat_x(1,1),y2_derivative_sampling,hat_x(2,1), mu_last, mu_p_last, u_last);
    else%在两个采样时刻之间
        predict_y=[1 0]*(A0*hat_x_last+B0*delta_u_last);
        hat_x=A_bar*hat_x_last + B_bar*delta_u_last/0.01+C_bar*predict_y_last;
        [u, delta_u, mu, mu_p]  = AIC2(t_now, 1, y_real,hat_x(1,1),y2_derivative_sampling,hat_x(2,1), mu_last, mu_p_last, u_last);
    end
end
end








% function [count,hat_x,predict_y, u, delta_u, mu, mu_p, mu_pp] = fcn(hat_x_last, predict_y_last, y_real,y2_derivative_sampling,y3_real_slow, u_last,delta_u_last,t_now,A_bar,B_bar,C_bar,A0,B0,mu_last, mu_p_last, mu_pp_last)
% if(t_now==0)
%     count=0;
%     hat_x = zeros(3,1);
%     predict_y = y_real;
%     hat_x(1,1)=y_real;
%     u_now=0;
%     hat_x = A_bar*hat_x + B_bar*u_now+ C_bar*predict_y;
%     [u, delta_u, mu, mu_p, mu_pp]  = AIC3(t_now, 1, y_real,hat_x(1,1),y2_derivative_sampling,hat_x(2,1), y3_real_slow, hat_x(3,1), mu_last, mu_p_last, mu_pp_last, u_last);
%     %predict_y=[1 0 0]*(A0*hat_x+B0*delta_u); 
%     
% else
%     count=mod(t_now,0.05);
%     if(count==0)%在采样的时刻
%         predict_y=y_real;
%         hat_x=A_bar*hat_x_last +B_bar*delta_u_last+ C_bar*predict_y;
%         %hat_x(1,1)=y_real;
%         [u, delta_u, mu, mu_p, mu_pp]  = AIC3(t_now, 1, y_real,hat_x(1,1),y2_derivative_sampling,hat_x(2,1), y3_real_slow, hat_x(3,1), mu_last, mu_p_last, mu_pp_last, u_last);
% 
%         %predict_y=[1 0 0]*(A0*hat_x+B0*delta_u);
%         
%     else%在两个采样时刻之间
%         predict_y=[1 0 0]*(A0*hat_x_last+B0*delta_u_last);
%         hat_x=A_bar*hat_x_last + B_bar*delta_u_last+C_bar*predict_y_last;
%         [u, delta_u, mu, mu_p, mu_pp]  = AIC3(t_now, 1, y_real,hat_x(1,1),y2_derivative_sampling,hat_x(2,1), y3_real_slow, hat_x(3,1), mu_last, mu_p_last, mu_pp_last, u_last);
%         %predict_y=[1 0 0]*(A0*hat_x+B0*delta_u);
%         
%     end
% end
% end

== matlab function ur5_simulink_ros2_pbvs_all_methods_2023b/RAID-AgIVS/Subsystem3/APO+AIC/MATLAB Function ==
  data: count output; hat_x_last input; predict_y_last input; y_real input; y2_derivative_sampling input; u_last input; delta_u_last input; hat_x output; t_now input; A_bar input; B_bar input; C_bar input; predict_y output; A0 input; B0 input; mu_last input; mu_p_last input; u output; delta_u output; mu output; mu_p output
function [count,hat_x,predict_y, u, delta_u, mu, mu_p] = fcn(hat_x_last, predict_y_last, y_real,y2_derivative_sampling, u_last,delta_u_last,t_now,A_bar,B_bar,C_bar,A0,B0,mu_last, mu_p_last)
if(t_now==0)
    count=0;
    hat_x = zeros(2,1);
    predict_y = y_real;
    hat_x(1,1)=y_real;
    [u, delta_u, mu, mu_p]  = AIC2(t_now, 1, y_real,hat_x(1,1),y2_derivative_sampling,hat_x(2,1), mu_last, mu_p_last, u_last);
else
    count=mod(t_now,0.05);
    if(count==0)%在采样的时刻
        predict_y=y_real;
        hat_x=A_bar*hat_x_last +B_bar*delta_u_last/0.01+ C_bar*predict_y;
        [u, delta_u, mu, mu_p]  = AIC2(t_now, 1, y_real,hat_x(1,1),y2_derivative_sampling,hat_x(2,1), mu_last, mu_p_last, u_last);
    else%在两个采样时刻之间
        predict_y=[1 0]*(A0*hat_x_last+B0*delta_u_last);
        hat_x=A_bar*hat_x_last + B_bar*delta_u_last/0.01+C_bar*predict_y_last;
        [u, delta_u, mu, mu_p]  = AIC2(t_now, 1, y_real,hat_x(1,1),y2_derivative_sampling,hat_x(2,1), mu_last, mu_p_last, u_last);
    end
end
end








% function [count,hat_x,predict_y, u, delta_u, mu, mu_p, mu_pp] = fcn(hat_x_last, predict_y_last, y_real,y2_derivative_sampling,y3_real_slow, u_last,delta_u_last,t_now,A_bar,B_bar,C_bar,A0,B0,mu_last, mu_p_last, mu_pp_last)
% if(t_now==0)
%     count=0;
%     hat_x = zeros(3,1);
%     predict_y = y_real;
%     hat_x(1,1)=y_real;
%     u_now=0;
%     hat_x = A_bar*hat_x + B_bar*u_now+ C_bar*predict_y;
%     [u, delta_u, mu, mu_p, mu_pp]  = AIC3(t_now, 1, y_real,hat_x(1,1),y2_derivative_sampling,hat_x(2,1), y3_real_slow, hat_x(3,1), mu_last, mu_p_last, mu_pp_last, u_last);
%     %predict_y=[1 0 0]*(A0*hat_x+B0*delta_u); 
%     
% else
%     count=mod(t_now,0.05);
%     if(count==0)%在采样的时刻
%         predict_y=y_real;
%         hat_x=A_bar*hat_x_last +B_bar*delta_u_last+ C_bar*predict_y;
%         %hat_x(1,1)=y_real;
%         [u, delta_u, mu, mu_p, mu_pp]  = AIC3(t_now, 1, y_real,hat_x(1,1),y2_derivative_sampling,hat_x(2,1), y3_real_slow, hat_x(3,1), mu_last, mu_p_last, mu_pp_last, u_last);
% 
%         %predict_y=[1 0 0]*(A0*hat_x+B0*delta_u);
%         
%     else%在两个采样时刻之间
%         predict_y=[1 0 0]*(A0*hat_x_last+B0*delta_u_last);
%         hat_x=A_bar*hat_x_last + B_bar*delta_u_last+C_bar*predict_y_last;
%         [u, delta_u, mu, mu_p, mu_pp]  = AIC3(t_now, 1, y_real,hat_x(1,1),y2_derivative_sampling,hat_x(2,1), y3_real_slow, hat_x(3,1), mu_last, mu_p_last, mu_pp_last, u_last);
%         %predict_y=[1 0 0]*(A0*hat_x+B0*delta_u);
%         
%     end
% end
% end

== matlab function ur5_simulink_ros2_pbvs_all_methods_2023b/MATLAB Function4 ==
  data: y output
function y = fcn()
    y =zeros(1,4);
    y(1) = 0.0;
    y(2) = 0.7071;
    y(3) = -0.7071;
    y(4) = 0.0;
end

== matlab function ur5_simulink_ros2_pbvs_all_methods_2023b/AIC/Subsystem2/AIC_muti_sensor_module/MATLAB Function ==
  data: u output; y1_real_slow input; y2_derivative_sampling input; mu output; mu_p output; mu_last input; mu_p_last input; u_last input
function [u, mu, mu_p]  = fcn(y1_real_slow,y2_derivative_sampling, mu_last, mu_p_last, u_last)
e_1=3;
e_2=3;
k_l=1;
sigma_z1_inv=0.2;
sigma_z2_inv=0.2;
sigma_w1_inv=1;
sigma_w2_inv=1;
k_i=-6;
k_p=-4.6;
T_c=0.05;
mu = double(mu_last + T_c*(mu_p_last+k_l*sigma_z1_inv*(y1_real_slow-mu_last)-k_l*sigma_w1_inv*e_1*(mu_p_last+e_1*mu_last)));
mu_p = double(mu_p_last + T_c*(k_l*sigma_z2_inv*(y2_derivative_sampling-mu_p_last)-k_l*sigma_w1_inv*(mu_p_last+e_1*mu_last)-k_l*sigma_w2_inv*e_2*e_2*mu_p_last));
u = double( u_last - T_c*(k_i*(y1_real_slow-mu)+k_p*(y2_derivative_sampling-mu_p)));
end

== matlab function ur5_simulink_ros2_pbvs_all_methods_2023b/MATLAB Function1 ==
  data: current_quat output; u input; y output; last_quat input
function [current_quat,y] = fcn(u, last_quat)
current_quat = u(4:7);
quat_dot = current_quat(1)*last_quat(1)+current_quat(2)*last_quat(2)+current_quat(3)*last_quat(3)++current_quat(4)*last_quat(4);
if(quat_dot<0)
    current_quat = -1*current_quat;
end
y = [u(1:3);current_quat];

== matlab function ur5_simulink_ros2_pbvs_all_methods_2023b/F-PID/Subsystem3/F-PID/MATLAB Function ==
  data: count output; hat_x_last input; y_real input; u_last input; hat_x output; t_now input; A_bar input; B_bar input; C_bar input; A0 input; B0 input
function [count, hat_x] = fcn(hat_x_last, y_real, u_last, t_now,A_bar,B_bar,C_bar,A0,B0)
if(t_now==0)
    count=0;
    hat_x = zeros(2,1);
    hat_x(1,1)=y_real;
else
    count=mod(t_now,0.05);
    if(count==0)%在采样的时刻
        hat_x=A_bar*hat_x_last +B_bar*u_last+ C_bar*y_real;
    else%在两个采样时刻之间
        hat_x = A0*hat_x_last+B0*u_last;
    end
end
end

% function [count,hat_x,predict_y, u, delta_u, mu, mu_p, mu_pp] = fcn(hat_x_last, predict_y_last, y_real,y2_derivative_sampling,y3_real_slow, u_last,delta_u_last,t_now,A_bar,B_bar,C_bar,A0,B0,mu_last, mu_p_last, mu_pp_last)
% if(t_now==0)
%     count=0;
%     hat_x = zeros(3,1);
%     predict_y = y_real;
%     hat_x(1,1)=y_real;
%     u_now=0;
%     hat_x = A_bar*hat_x + B_bar*u_now+ C_bar*predict_y;
%     [u, delta_u, mu, mu_p, mu_pp]  = AIC3(t_now, 1, y_real,hat_x(1,1),y2_derivative_sampling,hat_x(2,1), y3_real_slow, hat_x(3,1), mu_last, mu_p_last, mu_pp_last, u_last);
%     %predict_y=[1 0 0]*(A0*hat_x+B0*delta_u); 
%     
% else
%     count=mod(t_now,0.05);
%     if(count==0)%在采样的时刻
%         predict_y=y_real;
%         hat_x=A_bar*hat_x_last +B_bar*delta_u_last+ C_bar*predict_y;
%         %hat_x(1,1)=y_real;
%         [u, delta_u, mu, mu_p, mu_pp]  = AIC3(t_now, 1, y_real,hat_x(1,1),y2_derivative_sampling,hat_x(2,1), y3_real_slow, hat_x(3,1), mu_last, mu_p_last, mu_pp_last, u_last);
% 
%         %predict_y=[1 0 0]*(A0*hat_x+B0*delta_u);
%         
%     else%在两个采样时刻之间
%         predict_y=[1 0 0]*(A0*hat_x_last+B0*delta_u_last);
%         hat_x=A_bar*hat_x_last + B_bar*delta_u_last+C_bar*predict_y_last;
%         [u, delta_u, mu, mu_p, mu_pp]  = AIC3(t_now, 1, y_real,hat_x(1,1),y2_derivative_sampling,hat_x(2,1), y3_real_slow, hat_x(3,1), mu_last, mu_p_last, mu_pp_last, u_last);
%         %predict_y=[1 0 0]*(A0*hat_x+B0*delta_u);
%         
%     end
% end
% end

== matlab function ur5_simulink_ros2_pbvs_all_methods_2023b/Subsystem/MATLAB Function ==
  data: u input; x output; y output; z output
function [x,y,z]= fcn(u)
x = u(1);
y = u(2);
z = u(3);

== matlab function ur5_simulink_ros2_pbvs_all_methods_2023b/ROS2 Time Generator/MATLAB Function ==
  data: current_time input; last_time input; time_x output; init_time output
function [time_x,init_time] = fcn(current_time, last_time)
init_time = last_time;
time_x = current_time-last_time;

== matlab function ur5_simulink_ros2_pbvs_all_methods_2023b/Subsystem5/attitude_pi_ctrl/MATLAB Function ==
  data: R_current input; u output
function u  = attitudePIDControl(R_current)
    % 计算姿态误差矩阵
    Kp=0.9;

    % 在第一次调用时初始化
    % if isempty(isFirstCall)
    %     isFirstCall = false;
    %     R_target = R_current;  % 将当前姿态设置为目标姿态
    % end
    R_target=[0.7071,0.0001,0.7071,-0.0000];

    sym_ref = [0,-R_target(4),R_target(3);R_target(4),0,-R_target(2);-R_target(3),R_target(2),0];
    current_error_quat =R_current(1)*R_target(2:4)'-R_target(1)*R_current(2:4)'-sym_ref*R_current(2:4)';
    u=(Kp*current_error_quat); 
end

== matlab function ur5_simulink_ros2_pbvs_all_methods_2023b/AIC/Subsystem1/AIC_muti_sensor_module/MATLAB Function ==
  data: u output; y1_real_slow input; y2_derivative_sampling input; mu output; mu_p output; mu_last input; mu_p_last input; u_last input
function [u, mu, mu_p]  = fcn(y1_real_slow,y2_derivative_sampling, mu_last, mu_p_last, u_last)
e_1=3;
e_2=3;
k_l=1;
sigma_z1_inv=0.2;
sigma_z2_inv=0.2;
sigma_w1_inv=1;
sigma_w2_inv=1;
k_i=-6;
k_p=-4.6;
T_c=0.05;
mu = double(mu_last + T_c*(mu_p_last+k_l*sigma_z1_inv*(y1_real_slow-mu_last)-k_l*sigma_w1_inv*e_1*(mu_p_last+e_1*mu_last)));
mu_p = double(mu_p_last + T_c*(k_l*sigma_z2_inv*(y2_derivative_sampling-mu_p_last)-k_l*sigma_w1_inv*(mu_p_last+e_1*mu_last)-k_l*sigma_w2_inv*e_2*e_2*mu_p_last));
u = double( u_last - T_c*(k_i*(y1_real_slow-mu)+k_p*(y2_derivative_sampling-mu_p)));
end

== matlab function ur5_simulink_ros2_pbvs_all_methods_2023b/MATLAB Function ==
  data: Time_current input; flag output
function flag  = attitudePIDControl(Time_current)
    % if 0<Time_current && Time_current<6
    %     flag=4;
    % else
    %     if 6<=Time_current && Time_current<12
    %         flag=-4;
    %     else
    %         if 12<=Time_current && Time_current<18
    %             flag=4;
    %         else
    %             flag=-4;
    %         end
    %     end
    % end
    % if Time_current>=24
    %     flag=0;
    % end
    % 
    if 0<Time_current && Time_current<12
        flag=2;
    else
        if 12<=Time_current && Time_current<24
            flag=-2;
        else
            if 24<=Time_current && Time_current<36
                flag=2;
            else
                flag=-2;
            end
        end
    end
    if Time_current>=48
        flag=0;
    end

    % if 0<Time_current && Time_current<6
    %     flag=4;
    % else
    %     if 6<=Time_current && Time_current<18
    %         flag=-2;
    %     else
    %         if 18<=Time_current && Time_current<24
    %             flag=4;
    %         else
    %             flag=-2;
    %         end
    %     end
    % end
    % if Time_current>=55
    %     flag=0;
    % end

end

== matlab function ur5_simulink_ros2_pbvs_all_methods_2023b/PID Controller ==
  data: jacobian_matrix input; y output; current_error input
function y = fcn(jacobian_matrix, current_error)
    y = jacobian_matrix\current_error;
end

== matlab function ur5_simulink_ros2_pbvs_all_methods_2023b/AIC/Subsystem3/AIC_muti_sensor_module/MATLAB Function ==
  data: u output; y1_real_slow input; y2_derivative_sampling input; mu output; mu_p output; mu_last input; mu_p_last input; u_last input
function [u, mu, mu_p]  = fcn(y1_real_slow,y2_derivative_sampling, mu_last, mu_p_last, u_last)
e_1=3;
e_2=3;
k_l=1;
sigma_z1_inv=0.2;
sigma_z2_inv=0.2;
sigma_w1_inv=1;
sigma_w2_inv=1;
k_i=-6;
k_p=-4.6;
T_c=0.05;
mu = double(mu_last + T_c*(mu_p_last+k_l*sigma_z1_inv*(y1_real_slow-mu_last)-k_l*sigma_w1_inv*e_1*(mu_p_last+e_1*mu_last)));
mu_p = double(mu_p_last + T_c*(k_l*sigma_z2_inv*(y2_derivative_sampling-mu_p_last)-k_l*sigma_w1_inv*(mu_p_last+e_1*mu_last)-k_l*sigma_w2_inv*e_2*e_2*mu_p_last));
u = double( u_last - T_c*(k_i*(y1_real_slow-mu)+k_p*(y2_derivative_sampling-mu_p)));
end
